simulink model "FieldOrientedController_HIL"  (R2020b)
settings: configuration reference "SLRT_HIL" (kept outside this file)
undefined symbols (not defined in the file): encoderNumberOfSlits, idxVec, IO397, modeSchedulerEnum, pwmCounterMax, sampleTimeCurrentControl, velCmdVec
libraries: utils_lib x2, speedgoatlib_fpga_dio x2, simulink x2, SignalEditorBlockLib x1, speedgoatlib_interrupt x1, speedgoatlib_fpga_pwm x1, speedgoatlib_fpga_analog_io x1, speedgoatlib_fpga_inta x1, slrealtimetgmanagement x1, speedgoatlib_fpga_quadrature x1, speedgoatlib_fpga x1
settings Model: DataDictionary=mainData.sldd  EnableAccessToBaseWorkspace=off  SimulationMode=external  Creator=promero  LastModifiedBy=manuel.fedou
settings ConfigSetRef: SourceName=SLRT_HIL

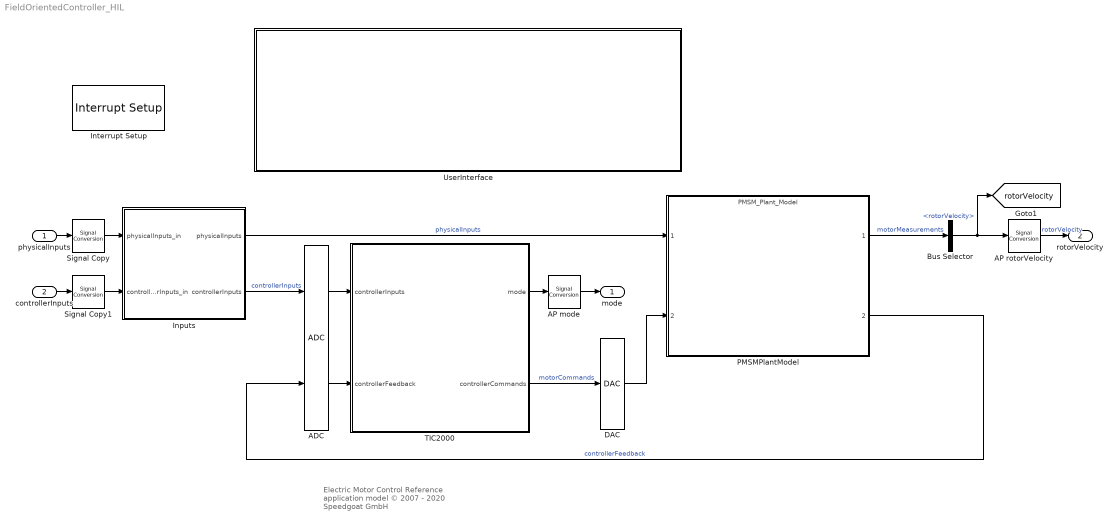
== system FieldOrientedController_HIL ==
  note: Electric Motor Control
      | Reference application model
      | © 2007 - 2020 Speedgoat GmbH
  physicalInputs : Inport  OutDataTypeStr=Bus: physicalInputs
  controllerInputs : Inport  Port=2  OutDataTypeStr=Bus: controllerInputs
  ADC : utils_lib/ADC  SystemSampleTime=-1  VariantActivationTime=update diagram  Latency=0  AutoFrameSizeCalculation=off
  AP mode : SignalConversion  OverrideOpt=off
  AP rotorVelocity : SignalConversion  OverrideOpt=off
  Bus Selector : BusSelector  OutputSignals=rotorVelocity
  DAC : utils_lib/DAC  SystemSampleTime=-1  VariantActivationTime=update diagram  Latency=0  AutoFrameSizeCalculation=off
  Inputs : Subsystem  Variant=on  VariantControlMode=label  VariantControl=Choice  LabelModeActiveChoice=dashboardInput
  Interrupt Setup : speedgoatlib_interrupt/Interrupt Setup  parModuleTrigger=on  parPollingMode=off  parPriorityConf=High  parPriority=241  confStartFcn=IO397_50k_v2_start_public  confStopFcn=IO397_50k_v2_stop_public  confIsrFcn=IO397_50k_v2_isr_public  confMapFcn=IO397_50k_v2_map_public  confHookFile=io397_50k_v2_int_hooks.c  confIrqNr=-1  confIsMdlTrig=on  confIsPolling=off  confPriority=254  confModID=1  confSelectedInt=Speedgoat IO397-50k v2 interrupt  confSelectedId=1
  PMSMPlantModel : ModelReference  ModelNameDialog=PMSM_Plant_Model  SimulationMode=Normal  ModelReferenceVersion=2.0
      mask Display: image('focVelocityEncoderMotorAndLoadAvgVoltageMask.png');
  Signal Copy : SignalConversion  OverrideOpt=off
  Signal Copy1 : SignalConversion  OverrideOpt=off
  TIC2000 : Subsystem  VariantControl=demoMode == 3
      mask Display: image('C2000.PNG');
  UserInterface : Subsystem
  mode : Outport
  rotorVelocity : Outport  Port=2
  tag scope: rotorVelocity=global
  wires:
  ADC/2 -> TIC2000/2(controllerFeedback)
  PMSMPlantModel/1 -> Bus Selector/1  "motorMeasurements"
  ADC/1 -> TIC2000/1(controllerInputs)
  TIC2000/2(" controllerCommands") -> DAC/1  "motorCommands"
  DAC/1 -> PMSMPlantModel/2
  Bus Selector/1 -> [rotorVelocity], AP rotorVelocity/1  "<rotorVelocity>"
  Inputs/2(controllerInputs) -> ADC/1  "controllerInputs"
  physicalInputs/1 -> Signal Copy/1
  controllerInputs/1 -> Signal Copy1/1
  Inputs/1(physicalInputs) -> PMSMPlantModel/1  "physicalInputs"
  AP rotorVelocity/1 -> rotorVelocity/1  "rotorVelocity"
  TIC2000/1(mode) -> AP mode/1
  AP mode/1 -> mode/1
  PMSMPlantModel/2 -> ADC/2  "controllerFeedback"
  Signal Copy/1 -> Inputs/1(physicalInputs_in)
  Signal Copy1/1 -> Inputs/2(controllerInputs_in)

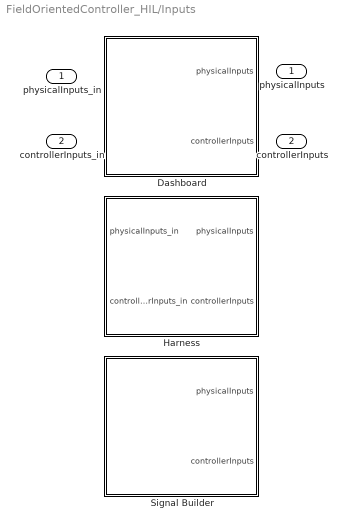
== system FieldOrientedController_HIL/Inputs ==
  physicalInputs_in : Inport  OutDataTypeStr=Bus: physicalInputs
  controllerInputs_in : Inport  Port=2  OutDataTypeStr=Bus: controllerInputs
  Dashboard : Subsystem  VariantControl=dashboardInput
  Harness : Subsystem  VariantControl=harnessInput
  Signal Builder : Subsystem  VariantControl=sigBuilderInput
  physicalInputs : Outport  OutDataTypeStr=Bus: physicalInputs
  controllerInputs : Outport  Port=2  OutDataTypeStr=Bus: controllerInputs

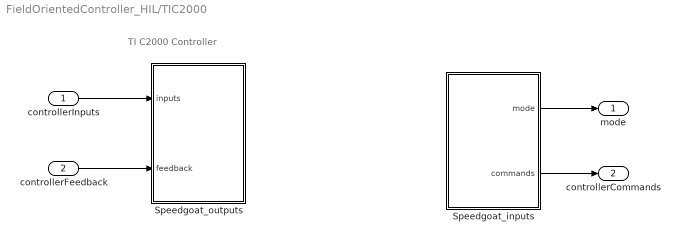
== system FieldOrientedController_HIL/TIC2000 ==
  note: TI C2000 Controller
  controllerInputs : Inport
  controllerFeedback : Inport  Port=2
  Speedgoat_inputs : Subsystem
  Speedgoat_outputs : Subsystem
  mode : Outport
  " controllerCommands" : Outport  Port=2  VectorParamsAs1DForOutWhenUnconnected=off
  wires:
  Speedgoat_inputs/2(commands) -> " controllerCommands"/1
  Speedgoat_inputs/1(mode) -> mode/1
  controllerFeedback/1 -> Speedgoat_outputs/2(feedback)
  controllerInputs/1 -> Speedgoat_outputs/1(inputs)

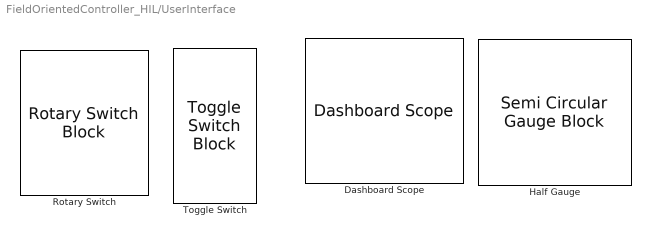
== system FieldOrientedController_HIL/UserInterface ==
  Dashboard Scope : DashboardScope  TimeSpan=10  Ymin=-200  Ymax=200  ScaleAtStop=off
  Half Gauge : SemiCircularGaugeBlock  ScaleMin=-200  ScaleMax=200
  Rotary Switch : RotarySwitchBlock
      settings: Values={{'-50', '0', '50', '100'}, [-50 0 50 100]}
  Toggle Switch : ToggleSwitchBlock
      settings: Values={{'Off', 'On'}, [0 1]}

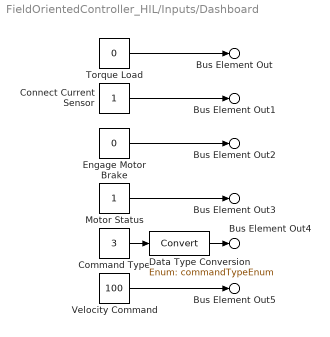
== system FieldOrientedController_HIL/Inputs/Dashboard ==
  Command Type : Constant  Value=3  OutDataTypeStr=uint8
  Connect Current Sensor : Constant  OutDataTypeStr=boolean
  Data Type Conversion : DataTypeConversion  OutDataTypeStr=Enum: commandTypeEnum
  Engage Motor Brake : Constant  Value=0  OutDataTypeStr=boolean
  Motor Status : Constant  OutDataTypeStr=boolean
  Torque Load : Constant  Value=0  OutDataTypeStr=Inherit: Inherit via back propagation
  Velocity Command : Constant  Value=100  OutDataTypeStr=Inherit: Inherit via back propagation
  Bus Element Out : Outport  PortName=physicalInputs  Element=torqueLoad
  Bus Element Out1 : Outport  PortName=physicalInputs  Element=connectCurrentSensor
  Bus Element Out2 : Outport  PortName=physicalInputs  Element=motorBrake
  Bus Element Out3 : Outport  Port=2  PortName=controllerInputs  Element=motorOn
  Bus Element Out4 : Outport  Port=2  PortName=controllerInputs  Element=commandType
  Bus Element Out5 : Outport  Port=2  PortName=controllerInputs  Element=velocityCommand
  wires:
  Engage Motor Brake/1 -> Bus Element Out2/1
  Data Type Conversion/1 -> Bus Element Out4/1
  Connect Current Sensor/1 -> Bus Element Out1/1
  Torque Load/1 -> Bus Element Out/1
  Velocity Command/1 -> Bus Element Out5/1
  Command Type/1 -> Data Type Conversion/1
  Motor Status/1 -> Bus Element Out3/1

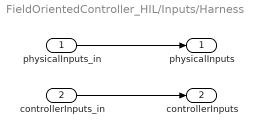
== system FieldOrientedController_HIL/Inputs/Harness ==
  physicalInputs_in : Inport  OutDataTypeStr=Bus: physicalInputs
  controllerInputs_in : Inport  Port=2  OutDataTypeStr=Bus: controllerInputs
  physicalInputs : Outport  OutDataTypeStr=Bus: physicalInputs
  controllerInputs : Outport  Port=2  OutDataTypeStr=Bus: controllerInputs
  wires:
  physicalInputs_in/1 -> physicalInputs/1
  controllerInputs_in/1 -> controllerInputs/1

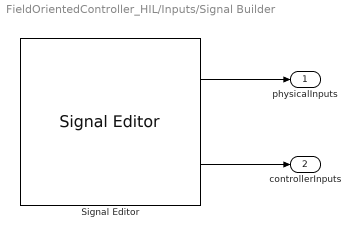
== system FieldOrientedController_HIL/Inputs/Signal Builder ==
  Signal Editor : SignalEditorBlockLib/Signal Editor  FileName=systemInputs.mat  ActiveScenario=doubleStepPosNegClosedLoop  ActiveSignal=controlInputs  IsBus=on  OutputBusObjectStr=Bus: controllerInputs  SampleTime=-1  Interpolate=off  ZeroCross=off  OutputAfterFinalValue=Holding final value  Unit=inherit  PreserveSignalName=on
  physicalInputs : Outport  OutDataTypeStr=Bus: physicalInputs
  controllerInputs : Outport  Port=2  OutDataTypeStr=Bus: controllerInputs
  wires:
  Signal Editor/1 -> physicalInputs/1
  Signal Editor/2 -> controllerInputs/1

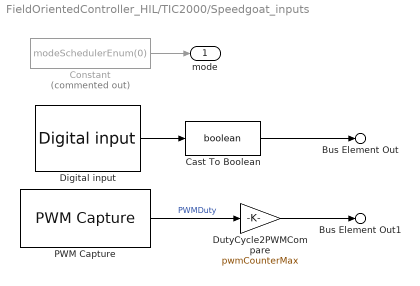
== system FieldOrientedController_HIL/TIC2000/Speedgoat_inputs ==
  Cast To Boolean : DataTypeConversion  OutDataTypeStr=boolean
  Constant : Constant  Commented=on  Value=modeSchedulerEnum(0)
  Digital input : speedgoatlib_fpga_dio/Digital input  id=1  chan=[2]  ts=sampleTimeCurrentControl  pciSlot=-1  board=IO397-50k  vectorizeOutput=off
      settings: SourceProductName=Simulink Real-Time: Speedgoat I/O Driver Library
  DutyCycle2PWMCompare : Gain  Gain=pwmCounterMax  OutDataTypeStr=Inherit: Inherit via back propagation
  PWM Capture : speedgoatlib_fpga_pwm/PWM Capture  id=1  chan=[1 2 3]  ts=sampleTimeCurrentControl  pciSlot=-1  board=IO397-50k  captureMode=High transitions triggered  captureTimeout=0  bit_width_cap=24  showHighDuration=off  showLowDuration=off  showPeriod=off  showDC16=on  showDC8=off  showTOn=off  showTOff=off  showValidData=off
      settings: SourceProductName=Simulink Real-Time: Speedgoat I/O Driver Library
  mode : Outport
  Bus Element Out : Outport  Port=2  PortName=commands  Element=inverterEnable
  Bus Element Out1 : Outport  Port=2  PortName=commands  Element=pwmCompare
  wires:
  PWM Capture/1 -> DutyCycle2PWMCompare/1  "PWMDuty"
  Digital input/1 -> Cast To Boolean/1
  DutyCycle2PWMCompare/1 -> Bus Element Out1/1
  Cast To Boolean/1 -> Bus Element Out/1
  Constant/1 -> mode/1

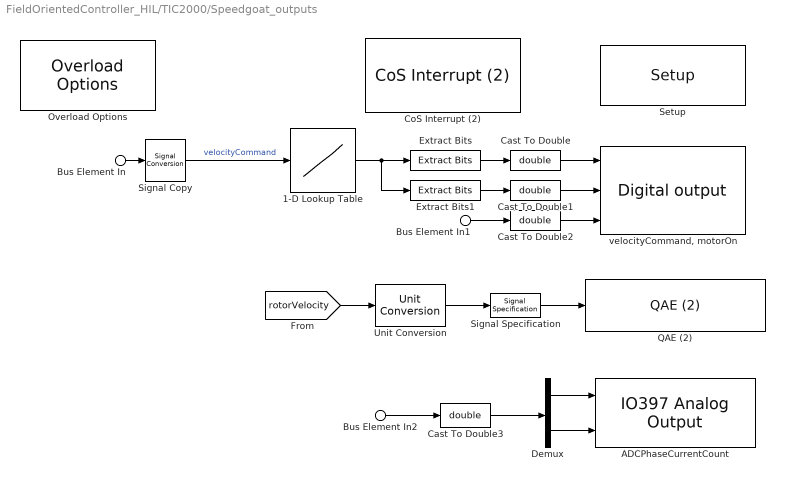
== system FieldOrientedController_HIL/TIC2000/Speedgoat_outputs ==
  Bus Element In1 : Inport  PortName=inputs  Element=motorOn
  Bus Element In : Inport  PortName=inputs  Element=velocityCommand
  Bus Element In2 : Inport  Port=2  PortName=feedback  Element=transducerVoltage
  1-D Lookup Table : Lookup_n-D  NumberOfTableDimensions=1  BreakpointsForDimension1=velCmdVec  Table=idxVec  InterpMethod=Flat  InternalRulePriority=Speed  OutDataTypeStr=uint8  RndMeth=Simplest  InputSameDT=on
  ADCPhaseCurrentCount : speedgoatlib_fpga_analog_io/IO397 Analog Output  id=1  chan=1:2  initVal=0  resetVal=1  ts=-1  pciSlot=-1  board=IO397-50k  span=+-5 V
      settings: SourceProductName=Simulink Real-Time: Speedgoat I/O Driver Library
  Cast To Double{,1..3} (4 alike) : DataTypeConversion  OutDataTypeStr=double
  CoS Interrupt (2) : speedgoatlib_fpga_inta/CoS Interrupt (2)  id=1  channel=[1]  pciSlot=-1  ts=-1  board=IO397-50k  fpga_frequency=0  int_source=internally generated  mode=0  debounce=0  delay=0  ad_settings=off  division=0  multiplication=0  gap=1e-3  int_freq=1/sampleTimeCurrentControl  freq_2_time=2.50000e-04  event=off  timestamp=off  flag=off
      settings: SourceProductName=Simulink Real-Time: Speedgoat Library
  Demux : Demux  Outputs=2
  Extract Bits : simulink/Logic and Bit Operations/Extract Bits  bitsToExtract=Range of bits  numBits=8  bitIdxRange=1  outScalingMode=Preserve fixed-point scaling
  Extract Bits1 : simulink/Logic and Bit Operations/Extract Bits  bitsToExtract=Range of bits  numBits=8  bitIdxRange=0  outScalingMode=Preserve fixed-point scaling
  Overload Options : slrealtimetgmanagement/Overload Options  startupDur=10  startupDurSrc=Tunable Parameter  maxOverload=10  maxOverloadSrc=Tunable Parameter  TETFlag=off
      settings: SourceProductBaseCode=XP
  QAE (2) : speedgoatlib_fpga_quadrature/QAE (2)  id=1  channel=1  ts=-1  pciSlot=-1  board=IO397-50k  numSeg=encoderNumberOfSlits*2  phaseAngle=90  initSpeed=0  initPos=pmsmRotorPositionInit  freeWheel=on  showInputSpeed=on  showInputPosition=off  showOutputPosition=off
      settings: SourceProductName=Simulink Real-Time: Speedgoat I/O Driver Library
  Setup : speedgoatlib_fpga/Setup/Setup  board=IO397-50k  id=1  device_id=1  frontIO=None  rearIO=None  bitstreamFile=speedgoat_IO397_50k_CI_02168  rev=1.0  timestamp_string=26/08/20 11:01:36  fpgaFreq=75 MHz  fpgaTick=13.33 ns  ProgSpiFlash=off  ProgBPIFlash=off  pciSlot=-1  PullRPort0=pull-up 3.3V  VioPort0=3.3V  PullRPort1=pull-up 3.3V  VioPort1=3.3V  PullRPort2=pull-up 3.3V  VioPort2=3.3V  PullRPort3=pull-up 3.3V  VioPort3=3.3V  PullRPort4=pull-up 3.3V  VioPort4=3.3V  PullRPort5=pull-up 3.3V  VioPort5=3.3V  PullRPort6=pull-up 3.3V  VioPort6=3.3V  PullRPort15=pull-up 3.3V  PullRPort31=pull-up 3.3V  PullRPort47=pull-up 3.3V  PullRPort63=pull-up 3.3V
      settings: SourceProductName=Simulink Real-Time: Speedgoat I/O Driver Library
  Signal Copy : SignalConversion  OverrideOpt=off
  Signal Specification : SignalSpecification  Unit=rpm
  Unit Conversion : UnitConversion
  "velocityCommand, motorOn" : speedgoatlib_fpga_dio/Digital output  id=1  chan=[3,4,1]  init=0  reset=1  vectorizeInput=off  ts=-1  pciSlot=-1  board=IO397-50k
      settings: SourceProductName=Simulink Real-Time: Speedgoat I/O Driver Library
  wires:
  Demux/2 -> ADCPhaseCurrentCount/2
  Demux/1 -> ADCPhaseCurrentCount/1
  1-D Lookup Table/1 -> Extract Bits1/1, Extract Bits/1
  Bus Element In1/1 -> Cast To Double2/1
  Cast To Double/1 -> "velocityCommand, motorOn"/1
  Cast To Double1/1 -> "velocityCommand, motorOn"/2
  Extract Bits/1 -> Cast To Double/1
  Extract Bits1/1 -> Cast To Double1/1
  Unit Conversion/1 -> Signal Specification/1
  Cast To Double2/1 -> "velocityCommand, motorOn"/3
  Cast To Double3/1 -> Demux/1
  Bus Element In/1 -> Signal Copy/1
  [rotorVelocity] -> Unit Conversion/1
  Signal Specification/1 -> QAE (2)/1
  Bus Element In2/1 -> Cast To Double3/1
  Signal Copy/1 -> 1-D Lookup Table/1  "velocityCommand"
